simulink model "TEST"  (R2014a)
settings: Solver=FixedStepDiscrete  SolverMode=SingleTasking  StartTime=0.0  StopTime=1  FixedStep=0.001  RelTol=1e-3  AbsTol=1e-6
Description:
  | Double to Fixed-Point Conversion
  | 
  | This model shows how to convert signals between built-in and
  | fixed-point data types and illustrates how fixed-point data types
  | affect the representable precision and range.  The fixed-point
  | data type used in this model is fixdt(1,5,2), which is a signed
  | 5-bit number with 2 bits to the right of the binary point:
  | 
  |    Precision = (2^-2) = 0.25
  |    Representable minimum = -(2^-2)*(2^4)   = -4
  |    Representable maximum =  (2^-2)*(2^4-1) = 3.75
  | 
  | Open the Data Type Conversion block 'Dbl-to-FixPt' to modify the
  | attributes of the fixed-point data type and see how they impact the
  | range and precision of the resulting fixed-point signal.
  | 
  | Tips for specifying fixed-point data types:
  | 
  | 
  | * Click the |>>| button to open the Data Type Assistant.
  | * You can specify the output minimum/maximum and use these
  | values to calculate the "best-precision scaling", which
  | maximizes the precision while covering the specified range.
  | * Once you are familiar with the syntax for fixdt, you can enter
  | the expression directly into the data type parameter without
  | using the Data Type Assistant.
settings Model: DataTypeOverride=Off  MinMaxOverflowLogging=MinMaxAndOverflow  CovMetricSettings=d  ExtModeTrigMode=oneshot  ExtModeArmWhenConnect=off  ExtModeAutoUpdateStatusClock=off  Creator=The MathWorks Inc.  LastModifiedBy=Caleb
settings DataIOCC: LimitDataPoints=off  SignalLoggingSaveFormat=ModelDataLogs  SignalLoggingName=sigsOut
settings OptimizationCC: BooleanDataType=off  ExpressionDepthLimit=2147483647  InitFltsAndDblsToZero=on
settings DebuggingCC: SignalRangeChecking=error  SaveWithParameterizedLinksMsg=none  UnderspecifiedInitializationDetection=Classic  SignalResolutionControl=TryResolveAllWithWarning  SolverPrmCheckMsg=none  MultiTaskDSMMsg=warning  MultiTaskCondExecSysMsg=none  SigSpecEnsureSampleTimeMsg=none  IntegerOverflowMsg=none  ParameterDowncastMsg=warning  ParameterOverflowMsg=warning  ParameterPrecisionLossMsg=none  FcnCallInpInsideContextMsg=UseLocalSettings  StateNameClashWarn=warning
settings HardwareCC: TargetUnknown=on
settings RTWCC: IncludeERTFirstTime=on
settings GRTTargetCC: TargetFcnLib=ansi_tfl_tmw.mat  CombineOutputUpdateFcns=off  GRTInterface=on

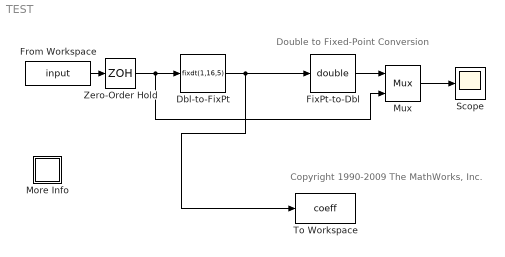
== system TEST ==
  note: Copyright 1990-2009 The MathWorks, Inc.
  note: Double to Fixed-Point Conversion
  Dbl-to-FixPt : DataTypeConversion  OutDataTypeStr=fixdt(1,16,5)
  FixPt-to-Dbl : DataTypeConversion  OutDataTypeStr=double
  From Workspace : FromWorkspace  VariableName=input  SampleTime=0
  More Info : Subsystem
      settings: OpenFcn=showdemo(bdroot(gcs))
      mask Display: disp('?')
  Mux : Mux  Inputs=2
  Scope : Scope
      settings: TickLabels=on  TimeRange=1  YMin=-10  YMax=10
  To Workspace : ToWorkspace  VariableName=coeff  SaveFormat=Timeseries  SampleTime=-1
  Zero-Order Hold : ZeroOrderHold  SampleTime=0.001
  wires:
  Zero-Order Hold/1 -> Mux/2, Dbl-to-FixPt/1
  From Workspace/1 -> Zero-Order Hold/1
  FixPt-to-Dbl/1 -> Mux/1
  Mux/1 -> Scope/1
  Dbl-to-FixPt/1 -> To Workspace/1, FixPt-to-Dbl/1

== system TEST/More Info ==
